simulink model "Subsystem"  (R2020b)
settings: Solver=VariableStepAuto  StartTime=0.0  StopTime=10.0  RelTol=1e-3
values from neighbouring files (symbols this model uses):
  ki = 40.0    [data.sldd]
  kp = 800.0    [data.sldd]
settings Model: DataDictionary=data.sldd  Creator=ANUJA  LastModifiedBy=ANUJA
settings DataIOCC: SaveOutput=off  SaveTime=off

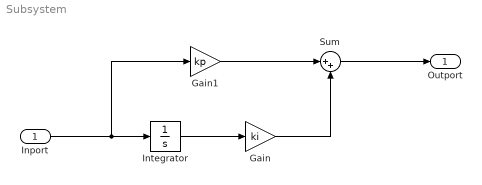
== system Subsystem ==
  Inport : Inport  OutDataTypeStr=double  PortDimensions=1  SampleTime=0
  Gain : Gain  Gain=ki
  Gain1 : Gain  Gain=kp
  Integrator : Integrator
  Sum : Sum  Inputs=|++
  Outport : Outport  OutDataTypeStr=double  PortDimensions=1  SampleTime=0
  wires:
  Gain/1 -> Sum/2
  Sum/1 -> Outport/1
  Inport/1 -> Gain1/1, Integrator/1
  Gain1/1 -> Sum/1
  Integrator/1 -> Gain/1
